simulink model "PIDControllerSimulink"  (R2020a)
settings: Solver=VariableStepAuto  StartTime=0.0  StopTime=10.0  RelTol=1e-3
values from neighbouring files (symbols this model uses):
  Kd = 1    [PIDControllerScript.m]
  Ki = 1    [PIDControllerScript.m]
  Kp = 2    [PIDControllerScript.m]
settings Model: Creator=diogo  LastModifiedBy=diogo

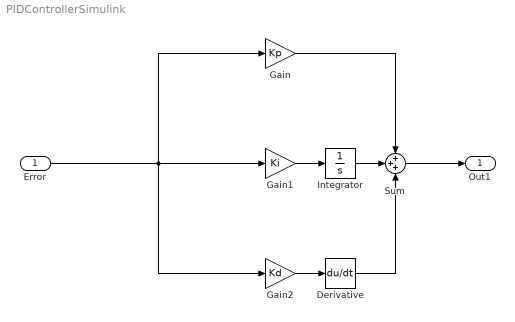
== system PIDControllerSimulink ==
  Error : Inport
  Derivative : Derivative
  Gain : Gain  Gain=Kp
  Gain1 : Gain  Gain=Ki
  Gain2 : Gain  Gain=Kd
  Integrator : Integrator
  Sum : Sum  Inputs=+++
  Out1 : Outport
  wires:
  Error/1 -> Gain1/1, Gain2/1, Gain/1
  Gain/1 -> Sum/1
  Gain1/1 -> Integrator/1
  Integrator/1 -> Sum/2
  Sum/1 -> Out1/1
  Gain2/1 -> Derivative/1
  Derivative/1 -> Sum/3
